simulink model "StateFlow_varB"  (R2022b)
settings: Solver=VariableStepAuto  StartTime=0.0  StopTime=500  FixedStep=0.001  RelTol=1e-3
InitFcn:
  | State_Flow_varB_setting
values from neighbouring files (symbols this model uses):
  Acceptable_press_offset = 5    [State_Flow_varB_setting.m]
  Desired_pressure_in_oxidiser_tank = 40    [State_Flow_varB_setting.m]
  Desired_pressure_in_pressure_section1 = 150    [State_Flow_varB_setting.m]
  Desired_pressure_in_pressure_section2 = 180    [State_Flow_varB_setting.m]
  s = struct    [State_Flow_varB_setting.m]
  Servo_open_limit = 20    [State_Flow_varB_setting.m]
  UDP_FC_send_packet_length = 68    [State_Flow_varB_setting.m]
  UDP_FC_send_sample_time = 0.05    [State_Flow_varB_setting.m]
  UDP_GSE_Curr_loop_receive_sample_time = 0.01    [State_Flow_varB_setting.m]
  UDP_GSE_IO_send_sample_time = 0.05    [State_Flow_varB_setting.m]
  UDP_GSE_send_packet_length = 68    [State_Flow_varB_setting.m]
libraries: simulink x36, slrealtimeiplib x16, slpidlib x6
(part 1 of 3)
settings Model: Creator=START  LastModifiedBy=START
settings DataIOCC: FinalStateName=xInitial  InitialState=SAVE  SaveOperatingPoint=on

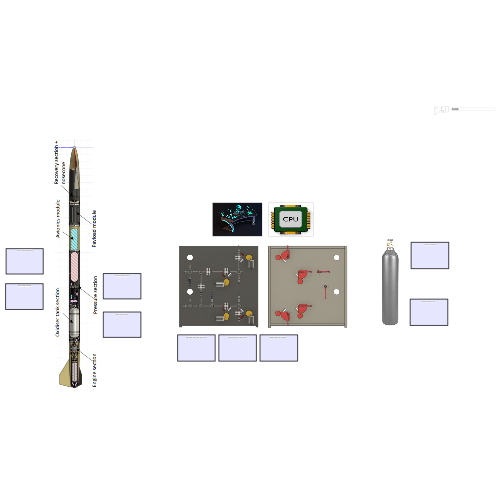
[thumbnail: Simulink's stored preview of the top-level diagram]
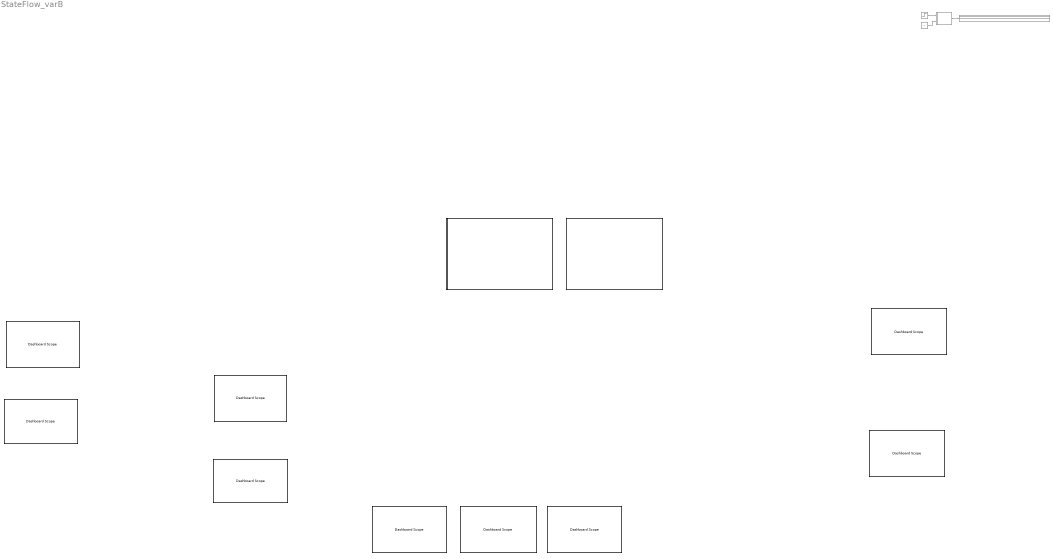
== system StateFlow_varB ==
  note: N2 bomb pressure level
  note: Rocket releasing valve state
  note: Rocket venting valve state
  note: Main tank pressure level
  note: Pressure section pressure level
  note: GSE N2 Releasing valve reported
  note: GSE N2 fueling valve state reported
  note: GSE Oxidiser fueling valve state reported
  note: N2O bomb pressure level
  Constant : Constant  Commented=on  Value=s  OutDataTypeStr=Bus: s_bus
  Dashboard Scope{,1,8,14} (4 alike) : DashboardScope  Ymin=0  Ymax=330
  Dashboard Scope11 : DashboardScope  Ymin=0  Ymax=260
  Dashboard Scope12 : DashboardScope  Ymin=0  Ymax=260
  Dashboard Scope13 : DashboardScope  Ymin=0  Ymax=260
  Dashboard Scope4 : DashboardScope  Ymin=0  Ymax=100
  Dashboard Scope6 : DashboardScope  Ymin=0  Ymax=90
  Display : Display  Commented=on
  MATLAB Function : MATLAB Function  Commented=on  TreatAsAtomicUnit=on
  Step : Step  Commented=on  SampleTime=0
  Subsystem4 : Subsystem
      mask Display: image('console4_1.jpg');
  Subsystem6 : Subsystem
      mask Display: image('CPU.png');
  wires:
  MATLAB Function/1(y) -> Display/1
  Step/1 -> MATLAB Function/1(u)
  Constant/1 -> MATLAB Function/2(inside)

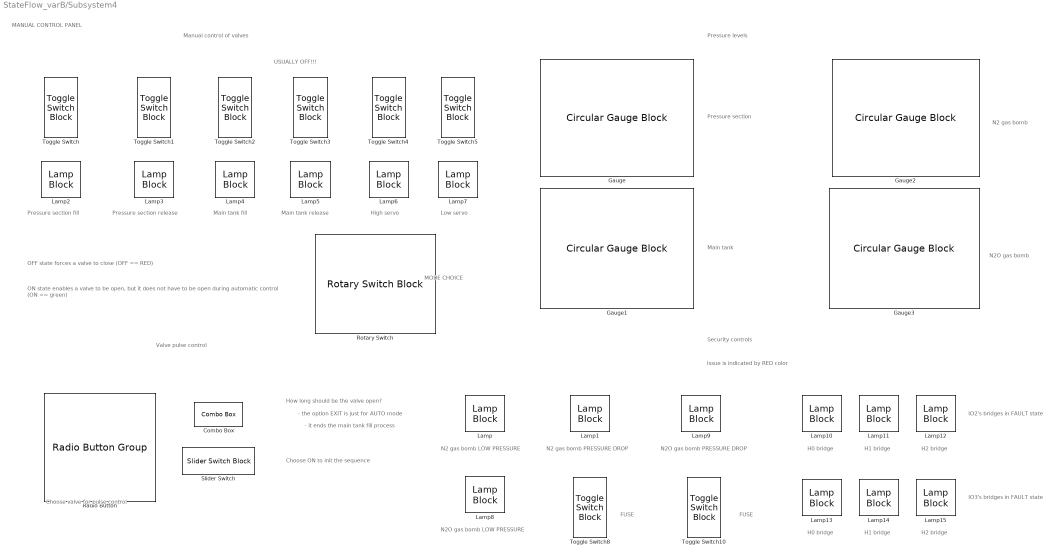
== system StateFlow_varB/Subsystem4 ==
  note: USUALLY OFF!!!
  note: N2 gas bomb LOW PRESSURE
  note: MANUAL CONTROL PANEL
  note: How long should be the valve open?
  note: Pressure levels
  note: Pressure section
  note: Main tank
  note: N2O gas bomb
  note: N2 gas bomb
  note: Manual control of valves
  note: Pressure section fill
  note: Pressure section release
  note: Main tank fill
  note: Main tank release
  note: High servo
  note: Low servo
  note: MODE CHOICE
  note: Security controls
  note: N2 gas bomb PRESSURE DROP
  note: OFF state forces a valve to close (OFF == RED)
  note: ON state enables a valve to be open, but it does not have to be open during automatic control (ON == green)
  note: N2O gas bomb LOW PRESSURE
  note: N2O gas bomb PRESSURE DROP
  note: Issue is indicated by RED color
  note: H0 bridge
  note: Valve pulse control
  note: - the option EXIT is just for AUTO mode
  note: - it ends the main tank fill process
  note: Choose ON to init the sequence
  note: Choose valve for pulse control
  note: FUSE
  note: FUSE
  note: IO2's bridges in FAULT state
  note: H1 bridge
  note: H2 bridge
  note: H1 bridge
  note: H2 bridge
  note: H0 bridge
  note: IO3's bridges in FAULT state
  Combo Box : ComboBox  LabelPosition=Hide  SelectedLabel=Exit
      settings: Values={{'0.5 s', '1 s', '2 s', '5 s', '10 s', 'Exit'}, [0 1 2 5 10 1000]}
  Gauge : CircularGaugeBlock  ScaleMax=300
  Gauge1 : CircularGaugeBlock
  Gauge2 : CircularGaugeBlock  ScaleMax=300
  Gauge3 : CircularGaugeBlock  ScaleMax=300
  Lamp{,1..15} (16 alike) : LampBlock  LabelPosition=Hide
  Radio Button : RadioButtonGroup  SelectedLabel=Main tank fill  ButtonGroupName=Valves
      settings: Values={{'Pressure section fill', 'Pressure section release', 'Main tank fill', 'Main tank release', 'High servo', 'Low servo'}, [0 1 2 3 4 5]}
  Rotary Switch : RotarySwitchBlock
      settings: Values={{'OFF', 'MAN', 'AUTO'}, [0 1 2]}
  Slider Switch : SliderSwitchBlock
      settings: Values={{'OFF', 'ON'}, [0 1]}
  Toggle Switch{,1..5,8,10} (8 alike) : ToggleSwitchBlock
      settings: Values={{'Off', 'On'}, [0 1]}

== system StateFlow_varB/Subsystem6 ==
  AND : Logic  IconShape=distinctive  AllPortsSameDT=off  OutDataTypeStr=boolean
  Chart : Stateflow chart  TreatAsAtomicUnit=on
  Compare To Constant : simulink/Logic and Bit Operations/Compare To Constant  relop===  const=1  OutDataTypeStr=boolean
  Compare To Constant1 : simulink/Logic and Bit Operations/Compare To Constant  relop===  const=2  OutDataTypeStr=boolean
  Constant : Constant  Value=2
  Constant1 : Constant
  Constant2 : Constant  Value=2
  Constant3 : Constant  Value=1000
  OR : Logic  Operator=OR  IconShape=distinctive  AllPortsSameDT=off  OutDataTypeStr=boolean
  Subsystem : Subsystem
  Subsystem1 : Subsystem
  Subsystem10 : Subsystem
  Subsystem2 : Subsystem
  Subsystem3 : Subsystem
  wires:
  Chart/1(AUTO_STATE) -> Subsystem/Enable
  Chart/2(MAN_STATE) -> Subsystem10/Enable
  Chart/3(OFF_STATE) -> Subsystem1/Enable
  Constant/1 -> Compare To Constant/1, Chart/1(CNTRL)
  Subsystem3/1(Output1) -> Subsystem/1(Input)
  Subsystem3/2(Input1) -> Subsystem/2(Input1)
  Subsystem3/3(Input2) -> Subsystem/3(Input2)
  Subsystem3/4(Input3) -> Subsystem/4(Input3)
  Subsystem3/5(Output) -> Subsystem/5(Input4)
  AND/1 -> Subsystem2/Enable
  OR/1 -> AND/1
  Constant1/1 -> Subsystem/7(Input6), AND/2
  Compare To Constant/1 -> OR/1
  Constant2/1 -> Subsystem2/1(Input), Compare To Constant1/1
  Compare To Constant1/1 -> OR/2
  Constant3/1 -> Subsystem/6(Input5), Subsystem2/2(Input1)

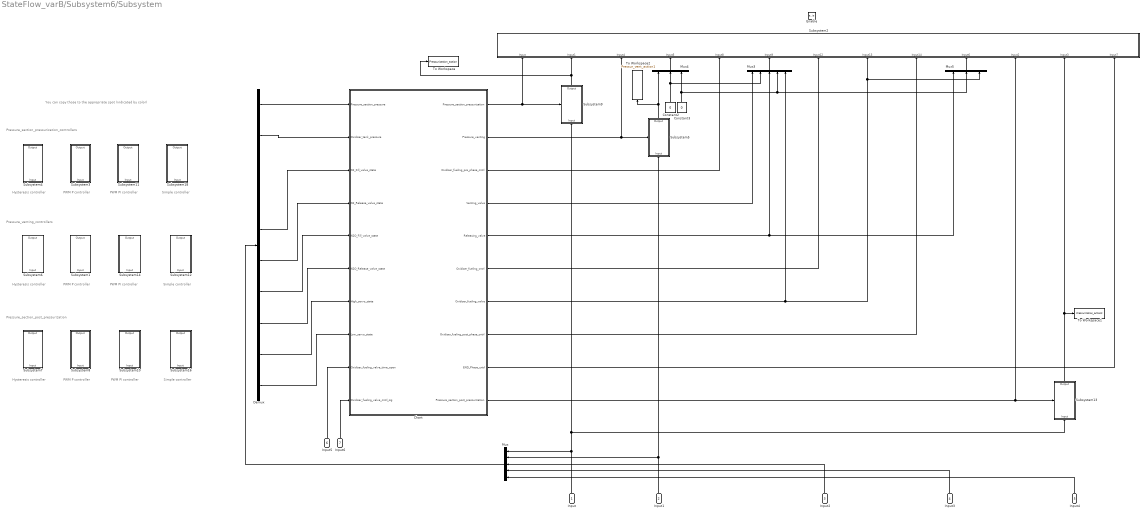
== system StateFlow_varB/Subsystem6/Subsystem ==
  note: You can copy those to the appropriate spot (indicated by color)
  note: Hysteresis controller
  note: Pressure_section_pressurization_controllers
  note: Hysteresis controller
  note: Pressure_venting_controllers
  note: Pressure_section_post_pressurization
  note: Hysteresis controller
  note: PWM P controller
  note: PWM P controller
  note: PWM PI controller
  note: PWM PI controller
  note: PWM P controller
  note: PWM PI controller
  note: Simple controller
  note: Simple controller
  note: Simple controller
  Input : Inport
  Input1 : Inport  Port=2
  Input2 : Inport  Port=3
  Input3 : Inport  Port=4
  Input4 : Inport  Port=5
  Input5 : Inport  Port=6
  Input6 : Inport  Port=7
  Enable : EnablePort  StatesWhenEnabling=reset
  Chart : Stateflow chart  TreatAsAtomicUnit=on
  Constant2 : Constant  Value=0
  Constant3 : Constant  Value=0
  Demux : Demux  Outputs=10
  Mux : Mux  Inputs=5
  Mux3 : Mux  Inputs=5
  Mux4 : Mux  Inputs=3
  Mux5 : Mux  Inputs=3
  Subsystem1 : Subsystem
  Subsystem10 : Subsystem
  Subsystem11 : Subsystem
  Subsystem12 : Subsystem
  Subsystem13 : Subsystem
  Subsystem14 : Subsystem
  Subsystem16 : Subsystem
  Subsystem18 : Subsystem
  Subsystem2 : Subsystem
  Subsystem3 : Subsystem
  Subsystem4 : Subsystem
  Subsystem5 : Subsystem
  Subsystem6 : Subsystem
  Subsystem7 : Subsystem
  Subsystem8 : Subsystem
  Subsystem9 : Subsystem
  To Workspace : ToWorkspace  VariableName=Pressurization_action  SaveFormat=Timeseries  SampleTime=-1
  To Workspace1 : ToWorkspace  VariableName=Pressurization_action2  SaveFormat=Timeseries  SampleTime=-1
  To Workspace2 : ToWorkspace  VariableName=Pressur_vent_action1  SaveFormat=Structure With Time  SampleTime=-1
  wires:
  Mux3/1 -> Subsystem2/6(Input9)
  Demux/10 -> Chart/8(Low_servo_state)
  Chart/7(Oxidiser_fueling_valve) -> Mux5/3, Subsystem2/8(Input13), Mux3/5
  Constant3/1 -> Mux5/2, Mux3/4, Mux4/3
  Chart/6(Oxidiser_fueling_cntrl) -> Subsystem2/7(Input12)
  Chart/3(Oxidiser_fueling_pre_phase_cntrl) -> Subsystem2/5(Input8)
  Input5/1 -> Chart/9(Oxidiser_fueling_valve_time_open)
  Demux/5 -> Chart/3(N2_Fill_valve_state)
  Chart/4(Venting_valve) -> Mux3/1
  Mux4/1 -> Subsystem2/4(Input5)
  Input/1 -> Mux/1, Subsystem13/1(Input), Subsystem9/1(Input)
  Constant2/1 -> Mux3/2, Mux4/2
  Input1/1 -> Subsystem5/1(Input), Mux/2
  Chart/2(Pressure_venting) -> Subsystem5/Enable, Subsystem2/3(Input4)
  Chart/5(Releasing_valve) -> Mux5/1, Mux3/3
  Subsystem9/1(Output) -> To Workspace/1, Subsystem2/2(Input1)
  Demux/1 -> Chart/1(Pressure_section_pressure)
  Input6/1 -> Chart/10(Oxidiser_fueling_valve_cntrl_sig)
  Mux/1 -> Demux/1
  Demux/2 -> Chart/2(Oxidiser_tank_pressure)
  Mux5/1 -> Subsystem2/10(Input6)
  Demux/7 -> Chart/5(N2O_Fill_valve_state)
  Demux/6 -> Chart/4(N2_Release_valve_state)
  Demux/9 -> Chart/7(High_servo_state)
  Demux/8 -> Chart/6(N2O_Release_valve_state)
  Subsystem5/1(Output) -> To Workspace2/1, Mux4/1
  Chart/8(Oxidiser_fueling_post_phase_cntrl) -> Subsystem2/9(Input14)
  Chart/9(END_Phase_cntrl) -> Subsystem2/13(Input7)
  Subsystem13/1(Output) -> To Workspace1/1, Subsystem2/12(Input3)
  Input2/1 -> Mux/3
  Input3/1 -> Mux/4
  Input4/1 -> Mux/5
  Chart/1(Pressure_section_pressurization) -> Subsystem9/Enable, Subsystem2/1(Input)
  Chart/10(Pressure_section_post_pressurization) -> Subsystem13/Enable, Subsystem2/11(Input2)

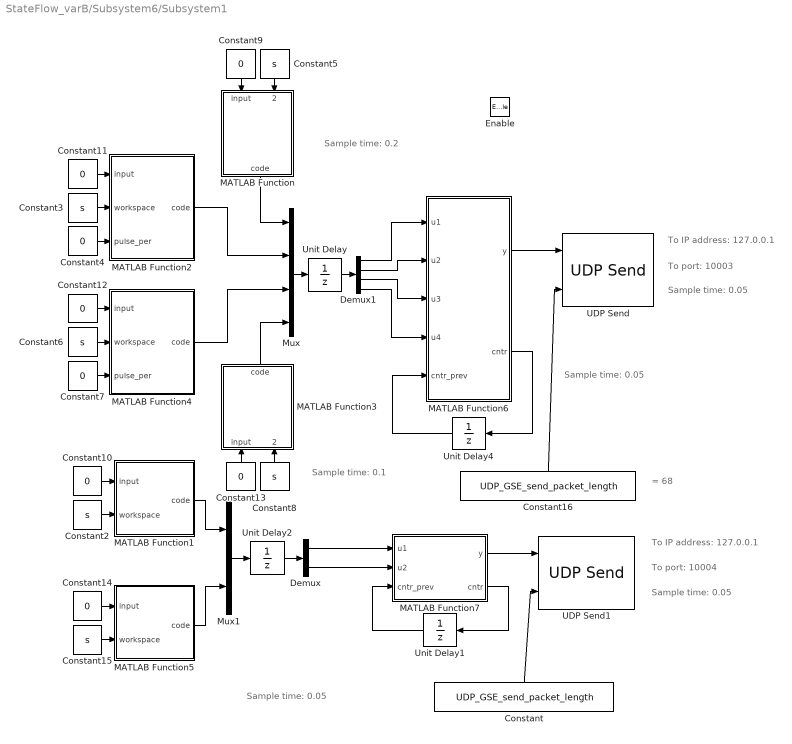
== system StateFlow_varB/Subsystem6/Subsystem1 ==
  note: To IP address: 127.0.0.1
  note: To port: 10003
  note: Sample time: 0.05
  note: To port: 10004
  note: To IP address: 127.0.0.1
  note: Sample time: 0.05
  note: = 68
  note: Sample time: 0.2
  note: Sample time: 0.05
  note: Sample time: 0.1
  note: Sample time: 0.05
  Enable : EnablePort  StatesWhenEnabling=reset
  Constant : Constant  Value=UDP_GSE_send_packet_length
  Constant{4,7,9..14} (8 alike) : Constant  Value=0
  Constant{2..3,5..6,8,15} (6 alike) : Constant  Value=s  OutDataTypeStr=Bus: s_bus
  Constant16 : Constant  Value=UDP_GSE_send_packet_length
  Demux : Demux  Outputs=2
  Demux1 : Demux
  MATLAB Function : MATLAB Function  TreatAsAtomicUnit=on
  MATLAB Function1 : MATLAB Function  TreatAsAtomicUnit=on
  MATLAB Function2 : MATLAB Function  TreatAsAtomicUnit=on
  MATLAB Function3 : MATLAB Function  TreatAsAtomicUnit=on
  MATLAB Function4 : MATLAB Function  TreatAsAtomicUnit=on
  MATLAB Function5 : MATLAB Function  TreatAsAtomicUnit=on
  MATLAB Function6 : MATLAB Function  TreatAsAtomicUnit=on
  MATLAB Function7 : MATLAB Function  TreatAsAtomicUnit=on
  Mux : Mux
  Mux1 : Mux  Inputs=2
  UDP Send : slrealtimeiplib/UDP Send  useHostTargetConn=off  toAddress=UDP_GSE_send_to_IP  toPort=IO_card_2_port  sampleTime=UDP_GSE_IO_send_sample_time  enableMessage=off
  UDP Send1 : slrealtimeiplib/UDP Send  useHostTargetConn=off  toAddress=UDP_GSE_send_to_IP  toPort=IO_card_3_port  sampleTime=UDP_GSE_IO_send_sample_time  enableMessage=off
  Unit Delay : UnitDelay  SampleTime=UDP_GSE_IO_send_sample_time*4  HasFrameUpgradeWarning=on
  Unit Delay1 : UnitDelay  InitialCondition=1  SampleTime=UDP_GSE_IO_send_sample_time  HasFrameUpgradeWarning=on
  Unit Delay2 : UnitDelay  SampleTime=UDP_GSE_IO_send_sample_time*2  HasFrameUpgradeWarning=on
  Unit Delay4 : UnitDelay  InitialCondition=1  SampleTime=UDP_GSE_IO_send_sample_time  HasFrameUpgradeWarning=on
  wires:
  Constant2/1 -> MATLAB Function1/2(workspace)
  Constant6/1 -> MATLAB Function4/2(workspace)
  Constant3/1 -> MATLAB Function2/2(workspace)
  Constant8/1 -> MATLAB Function3/2(workspace)
  Constant4/1 -> MATLAB Function2/3(pulse_per)
  Constant7/1 -> MATLAB Function4/3(pulse_per)
  Constant10/1 -> MATLAB Function1/1(input)
  Constant11/1 -> MATLAB Function2/1(input)
  Constant12/1 -> MATLAB Function4/1(input)
  Constant13/1 -> MATLAB Function3/1(input)
  Constant14/1 -> MATLAB Function5/1(input)
  Constant15/1 -> MATLAB Function5/2(workspace)
  Constant16/1 -> UDP Send/2
  MATLAB Function1/1(code) -> Mux1/1
  MATLAB Function5/1(code) -> Mux1/2
  Constant/1 -> UDP Send1/2
  Mux/1 -> Unit Delay/1
  MATLAB Function/1(code) -> Mux/1
  MATLAB Function2/1(code) -> Mux/2
  MATLAB Function4/1(code) -> Mux/3
  MATLAB Function3/1(code) -> Mux/4
  Mux1/1 -> Unit Delay2/1
  MATLAB Function7/2(cntr) -> Unit Delay1/1
  Unit Delay1/1 -> MATLAB Function7/3(cntr_prev)
  MATLAB Function7/1(y) -> UDP Send1/1
  Unit Delay2/1 -> Demux/1
  Demux/1 -> MATLAB Function7/1(u1)
  Demux/2 -> MATLAB Function7/2(u2)
  Unit Delay/1 -> Demux1/1
  Demux1/4 -> MATLAB Function6/4(u4)
  Demux1/3 -> MATLAB Function6/3(u3)
  MATLAB Function6/2(cntr) -> Unit Delay4/1
  Demux1/1 -> MATLAB Function6/1(u1)
  Unit Delay4/1 -> MATLAB Function6/5(cntr_prev)
  Demux1/2 -> MATLAB Function6/2(u2)
  MATLAB Function6/1(y) -> UDP Send/1
  Constant5/1 -> MATLAB Function/2(workspace)
  Constant9/1 -> MATLAB Function/1(input)

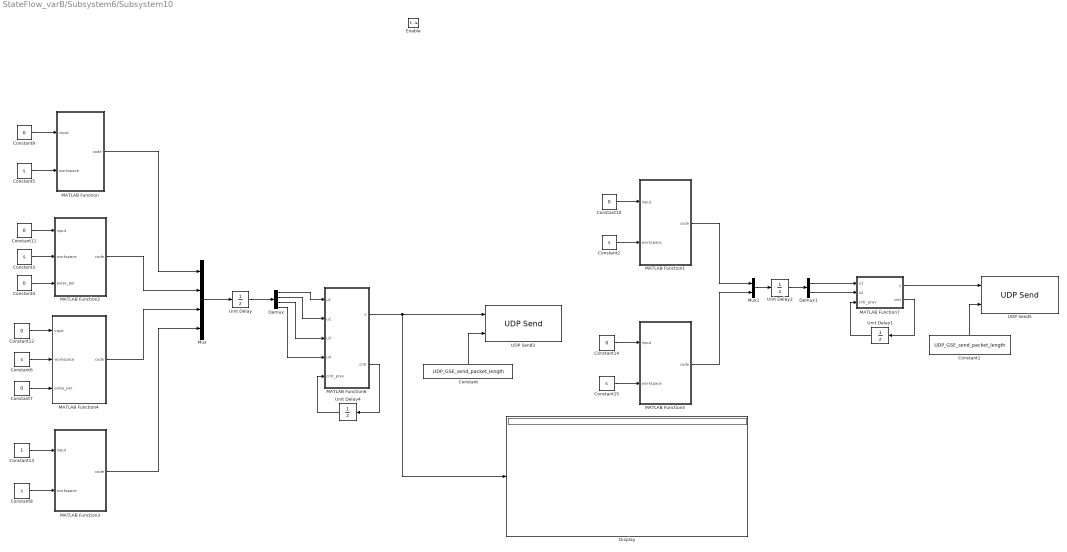
== system StateFlow_varB/Subsystem6/Subsystem10 ==
  Enable : EnablePort  StatesWhenEnabling=reset
  Constant : Constant  Value=UDP_GSE_send_packet_length
  Constant1 : Constant  Value=UDP_GSE_send_packet_length
  Constant{4,7,9..12,14} (7 alike) : Constant  Value=0
  Constant13 : Constant
  Constant{2..3,5..6,8,15} (6 alike) : Constant  Value=s  OutDataTypeStr=Bus: s_bus
  Demux : Demux
  Demux1 : Demux  Outputs=2
  Display : Display
  MATLAB Function : MATLAB Function  TreatAsAtomicUnit=on
  MATLAB Function1 : MATLAB Function  TreatAsAtomicUnit=on
  MATLAB Function2 : MATLAB Function  TreatAsAtomicUnit=on
  MATLAB Function3 : MATLAB Function  TreatAsAtomicUnit=on
  MATLAB Function4 : MATLAB Function  TreatAsAtomicUnit=on
  MATLAB Function5 : MATLAB Function  TreatAsAtomicUnit=on
  MATLAB Function6 : MATLAB Function  TreatAsAtomicUnit=on
  MATLAB Function7 : MATLAB Function  TreatAsAtomicUnit=on
  Mux : Mux
  Mux1 : Mux  Inputs=2
  UDP Send3 : slrealtimeiplib/UDP Send  useHostTargetConn=off  toAddress=UDP_GSE_send_to_IP  toPort=IO_card_2_port  sampleTime=UDP_GSE_IO_send_sample_time  enableMessage=off
  UDP Send5 : slrealtimeiplib/UDP Send  useHostTargetConn=off  toAddress=UDP_GSE_send_to_IP  toPort=IO_card_3_port  sampleTime=UDP_GSE_IO_send_sample_time  enableMessage=off
  Unit Delay : UnitDelay  SampleTime=UDP_GSE_IO_send_sample_time*4  HasFrameUpgradeWarning=on
  Unit Delay1 : UnitDelay  InitialCondition=1  SampleTime=UDP_GSE_IO_send_sample_time  HasFrameUpgradeWarning=on
  Unit Delay2 : UnitDelay  SampleTime=UDP_GSE_IO_send_sample_time*2  HasFrameUpgradeWarning=on
  Unit Delay4 : UnitDelay  InitialCondition=1  SampleTime=UDP_GSE_IO_send_sample_time  HasFrameUpgradeWarning=on
  wires:
  Constant2/1 -> MATLAB Function1/2(workspace)
  Constant6/1 -> MATLAB Function4/2(workspace)
  Constant3/1 -> MATLAB Function2/2(workspace)
  Constant8/1 -> MATLAB Function3/2(workspace)
  Constant4/1 -> MATLAB Function2/3(pulse_per)
  Constant7/1 -> MATLAB Function4/3(pulse_per)
  Constant10/1 -> MATLAB Function1/1(input)
  Constant11/1 -> MATLAB Function2/1(input)
  Constant12/1 -> MATLAB Function4/1(input)
  Constant13/1 -> MATLAB Function3/1(input)
  Constant14/1 -> MATLAB Function5/1(input)
  Constant15/1 -> MATLAB Function5/2(workspace)
  MATLAB Function/1(code) -> Mux/1
  Constant5/1 -> MATLAB Function/2(workspace)
  Constant9/1 -> MATLAB Function/1(input)
  MATLAB Function2/1(code) -> Mux/2
  MATLAB Function4/1(code) -> Mux/3
  MATLAB Function3/1(code) -> Mux/4
  Mux/1 -> Unit Delay/1
  MATLAB Function1/1(code) -> Mux1/1
  MATLAB Function5/1(code) -> Mux1/2
  Mux1/1 -> Unit Delay2/1
  Unit Delay/1 -> Demux/1
  Demux/4 -> MATLAB Function6/4(u4)
  Demux/3 -> MATLAB Function6/3(u3)
  MATLAB Function6/2(cntr) -> Unit Delay4/1
  Demux/1 -> MATLAB Function6/1(u1)
  Unit Delay4/1 -> MATLAB Function6/5(cntr_prev)
  Demux/2 -> MATLAB Function6/2(u2)
  Unit Delay2/1 -> Demux1/1
  MATLAB Function7/2(cntr) -> Unit Delay1/1
  Demux1/1 -> MATLAB Function7/1(u1)
  Unit Delay1/1 -> MATLAB Function7/3(cntr_prev)
  Demux1/2 -> MATLAB Function7/2(u2)
  MATLAB Function6/1(y) -> Display/1, UDP Send3/1
  Constant/1 -> UDP Send3/2
  MATLAB Function7/1(y) -> UDP Send5/1
  Constant1/1 -> UDP Send5/2

== system StateFlow_varB/Subsystem6/Subsystem2 ==
  Input : Inport
  Input1 : Inport  Port=2
  Enable : EnablePort  StatesWhenEnabling=reset
  MATLAB Function : MATLAB Function  TreatAsAtomicUnit=on
  Unit Delay : UnitDelay  SampleTime=0.05  HasFrameUpgradeWarning=on
  wires:
  Input/1 -> MATLAB Function/1(valve)
  Input1/1 -> MATLAB Function/2(time_des)
  MATLAB Function/1(time_curr) -> Unit Delay/1
  Unit Delay/1 -> MATLAB Function/3(time_curr1)

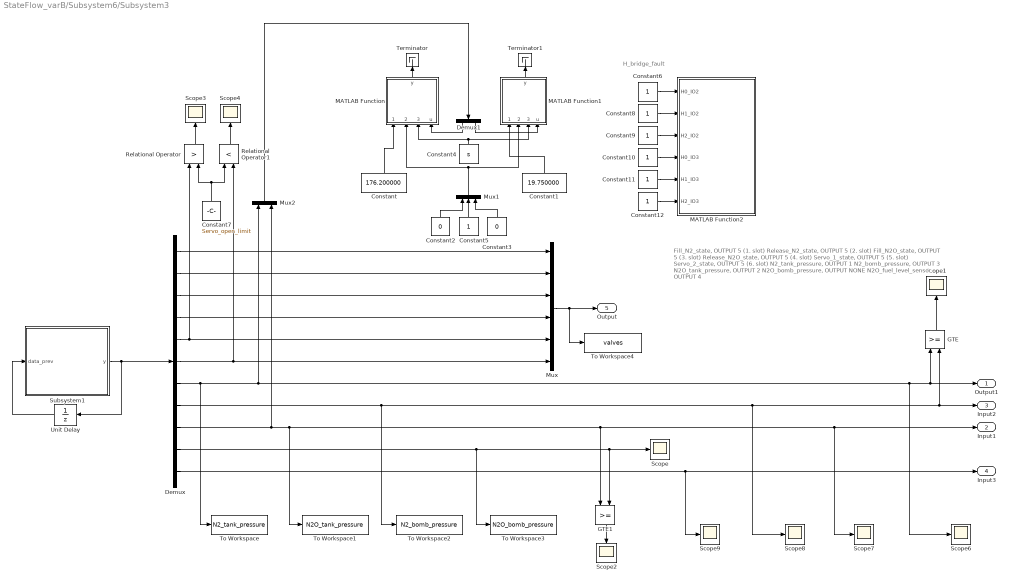
== system StateFlow_varB/Subsystem6/Subsystem3 ==
  note: H_bridge_fault
  note: Fill_N2_state, OUTPUT 5 (1. slot)
      | Release_N2_state, OUTPUT 5 (2. slot)
      | Fill_N2O_state, OUTPUT 5 (3. slot)
      | Release_N2O_state, OUTPUT 5 (4. slot)
      | Servo_1_state, OUTPUT 5 (5. slot)
      | Servo_2_state, OUTPUT 5 (6. slot)
      | N2_tank_pressure, OUTPUT 1
      | N2_bomb_pressure, OUTPUT 3
      | N2O_tank_pressure, OUTPUT 2
      | N2O_bomb_pressure, OUTPUT NONE
      | N2O_fuel_level_sensor OUTPUT 4
  Constant : Constant  Value=176.200000
  Constant1 : Constant  Value=19.750000
  Constant{5..6,8..12} (7 alike) : Constant
  Constant2 : Constant  Value=0
  Constant3 : Constant  Value=0
  Constant4 : Constant  Value=s  OutDataTypeStr=Bus: s_bus
  Constant7 : Constant  Value=Servo_open_limit
  Demux : Demux  Outputs=11
  Demux1 : Demux  Outputs=2
  GTE : RelationalOperator  OutDataTypeStr=boolean  RndMeth=Simplest  InputSameDT=off
  GTE1 : RelationalOperator  OutDataTypeStr=boolean  RndMeth=Simplest  InputSameDT=off
  MATLAB Function : MATLAB Function  TreatAsAtomicUnit=on
  MATLAB Function1 : MATLAB Function  TreatAsAtomicUnit=on
  MATLAB Function2 : MATLAB Function  TreatAsAtomicUnit=on
  Mux : Mux  Inputs=6
  Mux1 : Mux  Inputs=3
  Mux2 : Mux  Inputs=2
  Relational Operator : RelationalOperator  Operator=>  OutDataTypeStr=boolean  RndMeth=Simplest  InputSameDT=off
  Relational Operator1 : RelationalOperator  Operator=<  OutDataTypeStr=boolean  RndMeth=Simplest  InputSameDT=off
  Scope{,1..4,6..9} (9 alike) : Scope
  Subsystem1 : Subsystem
  Terminator : Terminator
  Terminator1 : Terminator
  To Workspace : ToWorkspace  VariableName=N2_tank_pressure  SaveFormat=Structure With Time  SampleTime=-1
  To Workspace1 : ToWorkspace  VariableName=N2O_tank_pressure  SaveFormat=Structure With Time  SampleTime=-1
  To Workspace2 : ToWorkspace  VariableName=N2_bomb_pressure  SaveFormat=Structure With Time  SampleTime=-1
  To Workspace3 : ToWorkspace  VariableName=N2O_bomb_pressure  SaveFormat=Structure With Time  SampleTime=-1
  To Workspace4 : ToWorkspace  VariableName=valves  SaveFormat=Structure With Time  SampleTime=-1
  Unit Delay : UnitDelay  SampleTime=-1  HasFrameUpgradeWarning=on
  Output1 : Outport
  Input1 : Outport  Port=2
  Input2 : Outport  Port=3
  Input3 : Outport  Port=4
  Output : Outport  Port=5
  wires:
  Subsystem1/1(y) -> Unit Delay/1, Demux/1
  Demux/7 -> To Workspace/1, Mux2/1, GTE/1, Output1/1, Scope6/1
  Demux/11 -> Scope9/1, Input3/1
  Demux/9 -> Mux2/2, To Workspace1/1, GTE1/1, Scope7/1, Input1/1
  Demux/8 -> To Workspace2/1, Scope8/1, GTE/2, Input2/1
  Demux/6 -> Relational Operator1/2, Mux/6
  Demux/5 -> Relational Operator/1, Mux/5
  Demux/4 -> Mux/4
  Demux/3 -> Mux/3
  Demux/2 -> Mux/2
  Demux/1 -> Mux/1
  Mux/1 -> To Workspace4/1, Output/1
  Unit Delay/1 -> Subsystem1/1(data_prev)
  Demux/10 -> To Workspace3/1, GTE1/2, Scope/1
  GTE/1 -> Scope1/1
  GTE1/1 -> Scope2/1
  Constant4/1 -> MATLAB Function/3(workspace), MATLAB Function1/3(workspace)
  MATLAB Function/1(y) -> Terminator/1
  Demux1/1 -> MATLAB Function/4(u)
  Constant/1 -> MATLAB Function/1(val_const)
  MATLAB Function1/1(y) -> Terminator1/1
  Mux1/1 -> MATLAB Function1/2(valves_state), MATLAB Function/2(valves_state)
  Demux1/2 -> MATLAB Function1/4(u)
  Constant1/1 -> MATLAB Function1/1(val_const)
  Constant2/1 -> Mux1/1
  Mux2/1 -> Demux1/1
  Constant5/1 -> Mux1/2
  Constant3/1 -> Mux1/3
  Constant6/1 -> MATLAB Function2/1(H0_IO2)
  Constant7/1 -> Relational Operator/2, Relational Operator1/1
  Relational Operator/1 -> Scope3/1
  Relational Operator1/1 -> Scope4/1
  Constant8/1 -> MATLAB Function2/2(H1_IO2)
  Constant9/1 -> MATLAB Function2/3(H2_IO2)
  Constant10/1 -> MATLAB Function2/4(H0_IO3)
  Constant11/1 -> MATLAB Function2/5(H1_IO3)
  Constant12/1 -> MATLAB Function2/6(H2_IO3)

== system StateFlow_varB/Subsystem6/Subsystem/Subsystem1 ==
  Input : Inport
  Enable : EnablePort
  Constant : Constant  Value=Desired_pressure_in_oxidiser_tank
  Constant1 : Constant  Commented=on  Value=s  OutDataTypeStr=Bus: s_bus
  Gain7 : Gain  Gain=-1
  MATLAB Function : MATLAB Function  Commented=on  TreatAsAtomicUnit=on
  Mux : Mux  Inputs=2
  PID Controller6 : slpidlib/PID Controller  Controller=PID  Form=Parallel  TimeDomain=Discrete-time  UseExternalTs=off  SampleTime=-1  IntegratorMethod=Forward Euler  FilterMethod=Forward Euler  ControllerParametersSource=internal  P=0.0077  I=0  UseKiTs=off  D=0  N=0  UseFilter=on  TunerSelectOption=Transfer Function Based (PID Tuner App)  InitialConditionSource=internal  InitialConditionForIntegrator=0  InitialConditionForFilter=0  DifferentiatorICPrevScaledInput=0  ExternalReset=none  TrackingMode=off  Kt=1  LimitOutput=on  SatLimitsSource=internal  UpperSaturationLimit=1  LowerSaturationLimit=-1  LinearizeAsGain=on  AntiWindupMode=clamping  Kb=1  LimitIntegrator=off  UpperIntegratorSaturationLimit=0.05  LowerIntegratorSaturationLimit=-inf  POutMin=[]  POutMax=[]  IOutMin=[]  IOutMax=[]  DOutMin=[]  DOutMax=[]  NOutMin=[]  NOutMax=[]  SumOutMin=[]  SumOutMax=[]  SaturationOutMin=[]  SaturationOutMax=[]  PParamMin=[]  PParamMax=[]  IParamMin=[]  IParamMax=[]  DParamMin=[]  DParamMax=[]  NParamMin=[]  NParamMax=[]  KbParamMin=[]  KbParamMax=[]  KtParamMin=[]  KtParamMax=[]  KbOutMin=[]  KbOutMax=[]  KtOutMin=[]  KtOutMax=[]  IntegratorOutMin=[]  IntegratorOutMax=[]  FilterOutMin=[]  FilterOutMax=[]  SumI1OutMin=[]  SumI1OutMax=[]  SumI2OutMin=[]  SumI2OutMax=[]  SumI3OutMin=[]  SumI3OutMax=[]  SumI4OutMin=[]  SumI4OutMax=[]  SumDOutMin=[]  SumDOutMax=[]  DifferentiatorOutMin=[]  DifferentiatorOutMax=[]  FilterDiffOutCoefMin=[]  FilterDiffOutCoefMax=[]  ReciprocalOutMin=[]  ReciprocalOutMax=[]  SumDenOutMin=[]  SumDenOutMax=[]  SumNumOutMin=[]  SumNumOutMax=[]  DivideOutMin=[]  DivideOutMax=[]  UdiffTsProdOutMin=[]  UdiffTsProdOutMax=[]  NTsProdOutMin=[]  NTsProdOutMax=[]  UintegralTsProdOutMin=[]  UintegralTsProdOutMax=[]  UngainTsProdOutMin=[]  UngainTsProdOutMax=[]  ClampingZeroOutDataTypeStr=Inherit: Inherit via back propagation  ClampingZeroOutMin=[]  ClampingZeroOutMax=[]  FilterDenConstantOutDataTypeStr=Inherit: Inherit via back propagation  FilterDenConstantOutMin=[]  FilterDenConstantOutMax=[]  PCopyOutDataTypeStr=Inherit: Inherit via back propagation  PCopyOutMin=[]  PCopyOutMax=[]  NCopyOutDataTypeStr=Inherit: Inherit via back propagation  NCopyOutMin=[]  NCopyOutMax=[]  IntegratorContinuousStateAttributes=''  IntegratorStateMustResolveToSignalObject=off  IntegratorRTWStateStorageClass=Auto  FilterContinuousStateAttributes=''  FilterStateMustResolveToSignalObject=off  FilterRTWStateStorageClass=Auto  ParallelPVariant=InternalParameters  IdealPVariant=Disabled  IVariant=InternalParameters  DVariant=InternalParameters  IntegratorVariant=Discrete  SatVariant=Enabled  AWVariant=DiscClampingParallel  PCopyVariant=Disabled  TRVariant=Disabled  FdbkBlocksVariant=Forward  IdealPFdbkVariant=Disabled  SatFdbkVariant=Disabled  DerivativeFilterVariant=ForwardEulerFilter  NVariant=InternalParameters  NCopyVariant=Disabled  FilterICVariant=InternalICsFilter  IntegratorICVariant=InternalICs  ExternalResetVariant=Disabled  TRSumVariant=Passthrough  SumFdbkVariant=Disabled  SumVariant=Sum_PID  TsampFilterVariant=InternalTs  TsampNgainVariant=Passthrough  TsampIntegralVariant=Passthrough  ExternalSaturationOutDataTypeStr=Inherit: Same as second input
  PWM : simulink/Discontinuities/PWM  DisableCoverage=on  Period=2  InitialDelay=0  DisallowZeroDutyCycle=off  RunAtFixedTimeIntervals=off  SampleTime=0.1
  PWM1 : simulink/Discontinuities/PWM  DisableCoverage=on  Period=2  InitialDelay=0  DisallowZeroDutyCycle=off  RunAtFixedTimeIntervals=off  SampleTime=0.1
  Sum8 : Sum  Inputs=|+-
  Terminator : Terminator  Commented=on
  Output : Outport
  wires:
  Constant/1 -> Sum8/1
  Sum8/1 -> PID Controller6/1
  PID Controller6/1 -> PWM/1, Gain7/1
  Gain7/1 -> PWM1/1
  Mux/1 -> Output/1
  Input/1 -> Sum8/2
  MATLAB Function/1(y) -> Terminator/1
  Constant1/1 -> MATLAB Function/3(workspace)
  PWM/1 -> Mux/1
  PWM1/1 -> Mux/2

== system StateFlow_varB/Subsystem6/Subsystem/Subsystem10 ==
  Input : Inport
  Enable : EnablePort
  Constant : Constant  Value=Desired_pressure_in_pressure_section1
  Gain4 : Gain  Gain=-1
  Mux : Mux  Inputs=2
  PID Controller5 : slpidlib/PID Controller  Controller=PID  Form=Parallel  TimeDomain=Discrete-time  UseExternalTs=off  SampleTime=-1  IntegratorMethod=Forward Euler  FilterMethod=Forward Euler  ControllerParametersSource=internal  P=0.0027  I=0.00002  UseKiTs=off  D=0  N=0  UseFilter=on  TunerSelectOption=Transfer Function Based (PID Tuner App)  InitialConditionSource=internal  InitialConditionForIntegrator=0  InitialConditionForFilter=0  DifferentiatorICPrevScaledInput=0  ExternalReset=none  TrackingMode=off  Kt=1  LimitOutput=on  SatLimitsSource=internal  UpperSaturationLimit=1  LowerSaturationLimit=-1  LinearizeAsGain=off  AntiWindupMode=clamping  Kb=1  LimitIntegrator=on  UpperIntegratorSaturationLimit=0.05  LowerIntegratorSaturationLimit=-0.05  POutMin=[]  POutMax=[]  IOutMin=[]  IOutMax=[]  DOutMin=[]  DOutMax=[]  NOutMin=[]  NOutMax=[]  SumOutMin=[]  SumOutMax=[]  SaturationOutMin=[]  SaturationOutMax=[]  PParamMin=[]  PParamMax=[]  IParamMin=[]  IParamMax=[]  DParamMin=[]  DParamMax=[]  NParamMin=[]  NParamMax=[]  KbParamMin=[]  KbParamMax=[]  KtParamMin=[]  KtParamMax=[]  KbOutMin=[]  KbOutMax=[]  KtOutMin=[]  KtOutMax=[]  IntegratorOutMin=[]  IntegratorOutMax=[]  FilterOutMin=[]  FilterOutMax=[]  SumI1OutMin=[]  SumI1OutMax=[]  SumI2OutMin=[]  SumI2OutMax=[]  SumI3OutMin=[]  SumI3OutMax=[]  SumI4OutMin=[]  SumI4OutMax=[]  SumDOutMin=[]  SumDOutMax=[]  DifferentiatorOutMin=[]  DifferentiatorOutMax=[]  FilterDiffOutCoefMin=[]  FilterDiffOutCoefMax=[]  ReciprocalOutMin=[]  ReciprocalOutMax=[]  SumDenOutMin=[]  SumDenOutMax=[]  SumNumOutMin=[]  SumNumOutMax=[]  DivideOutMin=[]  DivideOutMax=[]  UdiffTsProdOutMin=[]  UdiffTsProdOutMax=[]  NTsProdOutMin=[]  NTsProdOutMax=[]  UintegralTsProdOutMin=[]  UintegralTsProdOutMax=[]  UngainTsProdOutMin=[]  UngainTsProdOutMax=[]  ClampingZeroOutDataTypeStr=Inherit: Inherit via back propagation  ClampingZeroOutMin=[]  ClampingZeroOutMax=[]  FilterDenConstantOutDataTypeStr=Inherit: Inherit via back propagation  FilterDenConstantOutMin=[]  FilterDenConstantOutMax=[]  PCopyOutDataTypeStr=Inherit: Inherit via back propagation  PCopyOutMin=[]  PCopyOutMax=[]  NCopyOutDataTypeStr=Inherit: Inherit via back propagation  NCopyOutMin=[]  NCopyOutMax=[]  IntegratorContinuousStateAttributes=''  IntegratorStateMustResolveToSignalObject=off  IntegratorRTWStateStorageClass=Auto  FilterContinuousStateAttributes=''  FilterStateMustResolveToSignalObject=off  FilterRTWStateStorageClass=Auto  ParallelPVariant=InternalParameters  IdealPVariant=Disabled  IVariant=InternalParameters  DVariant=InternalParameters  IntegratorVariant=Discrete  SatVariant=Enabled  AWVariant=DiscClampingParallel  PCopyVariant=Disabled  TRVariant=Disabled  FdbkBlocksVariant=Forward  IdealPFdbkVariant=Disabled  SatFdbkVariant=Disabled  DerivativeFilterVariant=ForwardEulerFilter  NVariant=InternalParameters  NCopyVariant=Disabled  FilterICVariant=InternalICsFilter  IntegratorICVariant=InternalICs  ExternalResetVariant=Disabled  TRSumVariant=Passthrough  SumFdbkVariant=Disabled  SumVariant=Sum_PID  TsampFilterVariant=InternalTs  TsampNgainVariant=Passthrough  TsampIntegralVariant=Passthrough  ExternalSaturationOutDataTypeStr=Inherit: Same as second input
  PWM7 : simulink/Discontinuities/PWM  DisableCoverage=on  Period=2  InitialDelay=0  DisallowZeroDutyCycle=off  RunAtFixedTimeIntervals=off  SampleTime=0.1
  PWM8 : simulink/Discontinuities/PWM  DisableCoverage=on  Period=2  InitialDelay=0  DisallowZeroDutyCycle=off  RunAtFixedTimeIntervals=off  SampleTime=0.1
  Saturation13 : Saturate  UpperLimit=1  LowerLimit=0
  Saturation14 : Saturate  UpperLimit=1  LowerLimit=0
  Sum6 : Sum  Inputs=|+-
  Output : Outport
  wires:
  PID Controller5/1 -> Gain4/1, Saturation14/1
  Saturation13/1 -> PWM8/1
  Gain4/1 -> Saturation13/1
  Constant/1 -> Sum6/1
  Sum6/1 -> PID Controller5/1
  Saturation14/1 -> PWM7/1
  PWM8/1 -> Mux/2
  PWM7/1 -> Mux/1
  Mux/1 -> Output/1
  Input/1 -> Sum6/2

== system StateFlow_varB/Subsystem6/Subsystem/Subsystem11 ==
  Input : Inport
  Enable : EnablePort
  Constant : Constant  Value=Desired_pressure_in_pressure_section1
  Gain4 : Gain  Gain=-1
  Mux : Mux  Inputs=2
  PID Controller5 : slpidlib/PID Controller  Controller=PID  Form=Parallel  TimeDomain=Discrete-time  UseExternalTs=off  SampleTime=-1  IntegratorMethod=Forward Euler  FilterMethod=Forward Euler  ControllerParametersSource=internal  P=0.0027  I=0.00002  UseKiTs=off  D=0  N=0  UseFilter=on  TunerSelectOption=Transfer Function Based (PID Tuner App)  InitialConditionSource=internal  InitialConditionForIntegrator=0  InitialConditionForFilter=0  DifferentiatorICPrevScaledInput=0  ExternalReset=none  TrackingMode=off  Kt=1  LimitOutput=on  SatLimitsSource=internal  UpperSaturationLimit=1  LowerSaturationLimit=-1  LinearizeAsGain=off  AntiWindupMode=clamping  Kb=1  LimitIntegrator=on  UpperIntegratorSaturationLimit=0.05  LowerIntegratorSaturationLimit=-0.05  POutMin=[]  POutMax=[]  IOutMin=[]  IOutMax=[]  DOutMin=[]  DOutMax=[]  NOutMin=[]  NOutMax=[]  SumOutMin=[]  SumOutMax=[]  SaturationOutMin=[]  SaturationOutMax=[]  PParamMin=[]  PParamMax=[]  IParamMin=[]  IParamMax=[]  DParamMin=[]  DParamMax=[]  NParamMin=[]  NParamMax=[]  KbParamMin=[]  KbParamMax=[]  KtParamMin=[]  KtParamMax=[]  KbOutMin=[]  KbOutMax=[]  KtOutMin=[]  KtOutMax=[]  IntegratorOutMin=[]  IntegratorOutMax=[]  FilterOutMin=[]  FilterOutMax=[]  SumI1OutMin=[]  SumI1OutMax=[]  SumI2OutMin=[]  SumI2OutMax=[]  SumI3OutMin=[]  SumI3OutMax=[]  SumI4OutMin=[]  SumI4OutMax=[]  SumDOutMin=[]  SumDOutMax=[]  DifferentiatorOutMin=[]  DifferentiatorOutMax=[]  FilterDiffOutCoefMin=[]  FilterDiffOutCoefMax=[]  ReciprocalOutMin=[]  ReciprocalOutMax=[]  SumDenOutMin=[]  SumDenOutMax=[]  SumNumOutMin=[]  SumNumOutMax=[]  DivideOutMin=[]  DivideOutMax=[]  UdiffTsProdOutMin=[]  UdiffTsProdOutMax=[]  NTsProdOutMin=[]  NTsProdOutMax=[]  UintegralTsProdOutMin=[]  UintegralTsProdOutMax=[]  UngainTsProdOutMin=[]  UngainTsProdOutMax=[]  ClampingZeroOutDataTypeStr=Inherit: Inherit via back propagation  ClampingZeroOutMin=[]  ClampingZeroOutMax=[]  FilterDenConstantOutDataTypeStr=Inherit: Inherit via back propagation  FilterDenConstantOutMin=[]  FilterDenConstantOutMax=[]  PCopyOutDataTypeStr=Inherit: Inherit via back propagation  PCopyOutMin=[]  PCopyOutMax=[]  NCopyOutDataTypeStr=Inherit: Inherit via back propagation  NCopyOutMin=[]  NCopyOutMax=[]  IntegratorContinuousStateAttributes=''  IntegratorStateMustResolveToSignalObject=off  IntegratorRTWStateStorageClass=Auto  FilterContinuousStateAttributes=''  FilterStateMustResolveToSignalObject=off  FilterRTWStateStorageClass=Auto  ParallelPVariant=InternalParameters  IdealPVariant=Disabled  IVariant=InternalParameters  DVariant=InternalParameters  IntegratorVariant=Discrete  SatVariant=Enabled  AWVariant=DiscClampingParallel  PCopyVariant=Disabled  TRVariant=Disabled  FdbkBlocksVariant=Forward  IdealPFdbkVariant=Disabled  SatFdbkVariant=Disabled  DerivativeFilterVariant=ForwardEulerFilter  NVariant=InternalParameters  NCopyVariant=Disabled  FilterICVariant=InternalICsFilter  IntegratorICVariant=InternalICs  ExternalResetVariant=Disabled  TRSumVariant=Passthrough  SumFdbkVariant=Disabled  SumVariant=Sum_PID  TsampFilterVariant=InternalTs  TsampNgainVariant=Passthrough  TsampIntegralVariant=Passthrough  ExternalSaturationOutDataTypeStr=Inherit: Same as second input
  PWM7 : simulink/Discontinuities/PWM  DisableCoverage=on  Period=2  InitialDelay=0  DisallowZeroDutyCycle=off  RunAtFixedTimeIntervals=off  SampleTime=0.1
  PWM8 : simulink/Discontinuities/PWM  DisableCoverage=on  Period=2  InitialDelay=0  DisallowZeroDutyCycle=off  RunAtFixedTimeIntervals=off  SampleTime=0.1
  Saturation13 : Saturate  UpperLimit=1  LowerLimit=0
  Saturation14 : Saturate  UpperLimit=1  LowerLimit=0
  Sum6 : Sum  Inputs=|+-
  Output : Outport
  wires:
  PID Controller5/1 -> Gain4/1, Saturation14/1
  Saturation13/1 -> PWM8/1
  Gain4/1 -> Saturation13/1
  Constant/1 -> Sum6/1
  Sum6/1 -> PID Controller5/1
  Saturation14/1 -> PWM7/1
  PWM8/1 -> Mux/2
  PWM7/1 -> Mux/1
  Mux/1 -> Output/1
  Input/1 -> Sum6/2

== system StateFlow_varB/Subsystem6/Subsystem/Subsystem12 ==
  Input : Inport
  Enable : EnablePort
  Constant : Constant  Value=s  OutDataTypeStr=Bus: s_bus
  Constant1 : Constant  Value=Desired_pressure_in_oxidiser_tank
  MATLAB Function2 : MATLAB Function  TreatAsAtomicUnit=on
  Mux : Mux  Inputs=2
  PWM1 : simulink/Discontinuities/PWM  DisableCoverage=on  Period=2.5  InitialDelay=0  DisallowZeroDutyCycle=off  RunAtFixedTimeIntervals=off  SampleTime=0.1
  PWM2 : simulink/Discontinuities/PWM  DisableCoverage=on  Period=2.5  InitialDelay=0  DisallowZeroDutyCycle=off  RunAtFixedTimeIntervals=off  SampleTime=0.1
  Sum10 : Sum  Inputs=|+-
  Unit Delay : UnitDelay  InitialCondition=0.1  SampleTime=-1  HasFrameUpgradeWarning=on
  Unit Delay1 : UnitDelay  InitialCondition=Desired_pressure_in_oxidiser_tank-1  SampleTime=-1  HasFrameUpgradeWarning=on
  Output : Outport
  wires:
  Constant1/1 -> Sum10/1
  Sum10/1 -> Unit Delay1/1, MATLAB Function2/1(u)
  Constant/1 -> MATLAB Function2/3(workspace)
  Mux/1 -> Output/1
  Input/1 -> Sum10/2
  MATLAB Function2/3(duty) -> Unit Delay/1
  Unit Delay/1 -> MATLAB Function2/4(previous_duty)
  PWM1/1 -> Mux/1
  MATLAB Function2/1(fill) -> PWM1/1
  MATLAB Function2/2(release) -> PWM2/1
  PWM2/1 -> Mux/2
  Unit Delay1/1 -> MATLAB Function2/2(prev_u)

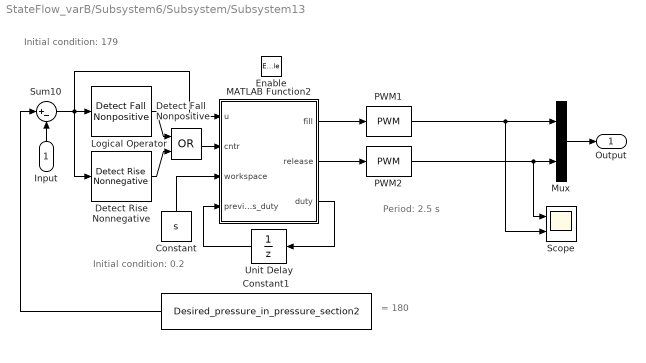
== system StateFlow_varB/Subsystem6/Subsystem/Subsystem13 ==
  note: Initial condition: 179
  note: Period: 2.5 s
  note: Initial condition: 0.2
  note: = 180
  Input : Inport
  Enable : EnablePort  StatesWhenEnabling=reset
  Constant : Constant  Value=s  OutDataTypeStr=Bus: s_bus
  Constant1 : Constant  Value=Desired_pressure_in_pressure_section2
  Detect Fall Nonpositive : simulink/Logic and Bit Operations/Detect Fall Nonpositive  vinit=Desired_pressure_in_pressure_section2 - 1  OutDataTypeStr=boolean
  Detect Rise Nonnegative : simulink/Logic and Bit Operations/Detect Rise Nonnegative  vinit=Desired_pressure_in_pressure_section2-1  OutDataTypeStr=boolean
  Logical Operator : Logic  Operator=OR  AllPortsSameDT=off  OutDataTypeStr=boolean
  MATLAB Function2 : MATLAB Function  TreatAsAtomicUnit=on
  Mux : Mux  Inputs=2
  PWM1 : simulink/Discontinuities/PWM  DisableCoverage=on  Period=2.5  InitialDelay=0  DisallowZeroDutyCycle=off  RunAtFixedTimeIntervals=off  SampleTime=0.1
  PWM2 : simulink/Discontinuities/PWM  DisableCoverage=on  Period=2.5  InitialDelay=0  DisallowZeroDutyCycle=off  RunAtFixedTimeIntervals=off  SampleTime=0.1
  Scope : Scope  NumInputPorts=2
  Sum10 : Sum  Inputs=|+-
  Unit Delay : UnitDelay  InitialCondition=0.2  SampleTime=-1  HasFrameUpgradeWarning=on
  Output : Outport
  wires:
  Logical Operator/1 -> MATLAB Function2/2(cntr)
  Detect Fall Nonpositive/1 -> Logical Operator/1
  Detect Rise Nonnegative/1 -> Logical Operator/2
  PWM2/1 -> Scope/1, Mux/2
  MATLAB Function2/2(release) -> PWM2/1
  MATLAB Function2/1(fill) -> PWM1/1
  PWM1/1 -> Scope/2, Mux/1
  Unit Delay/1 -> MATLAB Function2/4(previous_duty)
  MATLAB Function2/3(duty) -> Unit Delay/1
  Input/1 -> Sum10/2
  Mux/1 -> Output/1
  Constant/1 -> MATLAB Function2/3(workspace)
  Sum10/1 -> Detect Fall Nonpositive/1, MATLAB Function2/1(u), Detect Rise Nonnegative/1
  Constant1/1 -> Sum10/1

== system StateFlow_varB/Subsystem6/Subsystem/Subsystem14 ==
  Input : Inport
  Enable : EnablePort
  Constant : Constant  Value=Desired_pressure_in_oxidiser_tank
  Constant1 : Constant  Commented=on  Value=s  OutDataTypeStr=Bus: s_bus
  Gain5 : Gain  Gain=-1
  MATLAB Function : MATLAB Function  Commented=on  TreatAsAtomicUnit=on
  Mux : Mux  Inputs=2
  PID Controller7 : slpidlib/PID Controller  Controller=PID  Form=Parallel  TimeDomain=Discrete-time  UseExternalTs=off  SampleTime=-1  IntegratorMethod=Forward Euler  FilterMethod=Forward Euler  ControllerParametersSource=internal  P=0.008  I=0.00068  UseKiTs=off  D=0  N=0  UseFilter=on  TunerSelectOption=Transfer Function Based (PID Tuner App)  InitialConditionSource=internal  InitialConditionForIntegrator=0  InitialConditionForFilter=0  DifferentiatorICPrevScaledInput=0  ExternalReset=none  TrackingMode=off  Kt=1  LimitOutput=on  SatLimitsSource=internal  UpperSaturationLimit=1  LowerSaturationLimit=-1  LinearizeAsGain=off  AntiWindupMode=clamping  Kb=1  LimitIntegrator=on  UpperIntegratorSaturationLimit=1  LowerIntegratorSaturationLimit=-1  POutMin=[]  POutMax=[]  IOutMin=[]  IOutMax=[]  DOutMin=[]  DOutMax=[]  NOutMin=[]  NOutMax=[]  SumOutMin=[]  SumOutMax=[]  SaturationOutMin=[]  SaturationOutMax=[]  PParamMin=[]  PParamMax=[]  IParamMin=[]  IParamMax=[]  DParamMin=[]  DParamMax=[]  NParamMin=[]  NParamMax=[]  KbParamMin=[]  KbParamMax=[]  KtParamMin=[]  KtParamMax=[]  KbOutMin=[]  KbOutMax=[]  KtOutMin=[]  KtOutMax=[]  IntegratorOutMin=[]  IntegratorOutMax=[]  FilterOutMin=[]  FilterOutMax=[]  SumI1OutMin=[]  SumI1OutMax=[]  SumI2OutMin=[]  SumI2OutMax=[]  SumI3OutMin=[]  SumI3OutMax=[]  SumI4OutMin=[]  SumI4OutMax=[]  SumDOutMin=[]  SumDOutMax=[]  DifferentiatorOutMin=[]  DifferentiatorOutMax=[]  FilterDiffOutCoefMin=[]  FilterDiffOutCoefMax=[]  ReciprocalOutMin=[]  ReciprocalOutMax=[]  SumDenOutMin=[]  SumDenOutMax=[]  SumNumOutMin=[]  SumNumOutMax=[]  DivideOutMin=[]  DivideOutMax=[]  UdiffTsProdOutMin=[]  UdiffTsProdOutMax=[]  NTsProdOutMin=[]  NTsProdOutMax=[]  UintegralTsProdOutMin=[]  UintegralTsProdOutMax=[]  UngainTsProdOutMin=[]  UngainTsProdOutMax=[]  ClampingZeroOutDataTypeStr=Inherit: Inherit via back propagation  ClampingZeroOutMin=[]  ClampingZeroOutMax=[]  FilterDenConstantOutDataTypeStr=Inherit: Inherit via back propagation  FilterDenConstantOutMin=[]  FilterDenConstantOutMax=[]  PCopyOutDataTypeStr=Inherit: Inherit via back propagation  PCopyOutMin=[]  PCopyOutMax=[]  NCopyOutDataTypeStr=Inherit: Inherit via back propagation  NCopyOutMin=[]  NCopyOutMax=[]  IntegratorContinuousStateAttributes=''  IntegratorStateMustResolveToSignalObject=off  IntegratorRTWStateStorageClass=Auto  FilterContinuousStateAttributes=''  FilterStateMustResolveToSignalObject=off  FilterRTWStateStorageClass=Auto  ParallelPVariant=InternalParameters  IdealPVariant=Disabled  IVariant=InternalParameters  DVariant=InternalParameters  IntegratorVariant=Discrete  SatVariant=Enabled  AWVariant=DiscClampingParallel  PCopyVariant=Disabled  TRVariant=Disabled  FdbkBlocksVariant=Forward  IdealPFdbkVariant=Disabled  SatFdbkVariant=Disabled  DerivativeFilterVariant=ForwardEulerFilter  NVariant=InternalParameters  NCopyVariant=Disabled  FilterICVariant=InternalICsFilter  IntegratorICVariant=InternalICs  ExternalResetVariant=Disabled  TRSumVariant=Passthrough  SumFdbkVariant=Disabled  SumVariant=Sum_PID  TsampFilterVariant=InternalTs  TsampNgainVariant=Passthrough  TsampIntegralVariant=Passthrough  ExternalSaturationOutDataTypeStr=Inherit: Same as second input
  PWM : simulink/Discontinuities/PWM  DisableCoverage=on  Period=2  InitialDelay=0  DisallowZeroDutyCycle=off  RunAtFixedTimeIntervals=off  SampleTime=0.1
  PWM1 : simulink/Discontinuities/PWM  DisableCoverage=on  Period=2  InitialDelay=0  DisallowZeroDutyCycle=off  RunAtFixedTimeIntervals=off  SampleTime=0.1
  Sum9 : Sum  Inputs=|+-
  Terminator : Terminator  Commented=on
  Output : Outport
  wires:
  Constant/1 -> Sum9/1
  Sum9/1 -> PID Controller7/1
  PID Controller7/1 -> PWM/1, Gain5/1
  PWM/1 -> Mux/1
  Gain5/1 -> PWM1/1
  Input/1 -> Sum9/2
  Mux/1 -> Output/1
  MATLAB Function/1(y) -> Terminator/1
  Constant1/1 -> MATLAB Function/3(workspace)
  PWM1/1 -> Mux/2

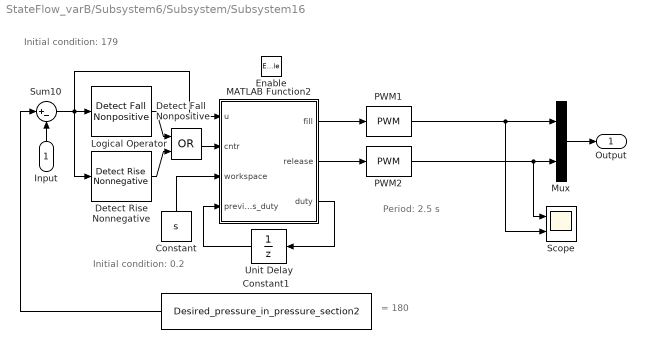
== system StateFlow_varB/Subsystem6/Subsystem/Subsystem16 ==
  note: Initial condition: 179
  note: Period: 2.5 s
  note: Initial condition: 0.2
  note: = 180
  Input : Inport
  Enable : EnablePort  StatesWhenEnabling=reset
  Constant : Constant  Value=s  OutDataTypeStr=Bus: s_bus
  Constant1 : Constant  Value=Desired_pressure_in_pressure_section2
  Detect Fall Nonpositive : simulink/Logic and Bit Operations/Detect Fall Nonpositive  vinit=Desired_pressure_in_pressure_section2 - 1  OutDataTypeStr=boolean
  Detect Rise Nonnegative : simulink/Logic and Bit Operations/Detect Rise Nonnegative  vinit=Desired_pressure_in_pressure_section2-1  OutDataTypeStr=boolean
  Logical Operator : Logic  Operator=OR  AllPortsSameDT=off  OutDataTypeStr=boolean
  MATLAB Function2 : MATLAB Function  TreatAsAtomicUnit=on
  Mux : Mux  Inputs=2
  PWM1 : simulink/Discontinuities/PWM  DisableCoverage=on  Period=2.5  InitialDelay=0  DisallowZeroDutyCycle=off  RunAtFixedTimeIntervals=off  SampleTime=0.1
  PWM2 : simulink/Discontinuities/PWM  DisableCoverage=on  Period=2.5  InitialDelay=0  DisallowZeroDutyCycle=off  RunAtFixedTimeIntervals=off  SampleTime=0.1
  Scope : Scope  NumInputPorts=2
  Sum10 : Sum  Inputs=|+-
  Unit Delay : UnitDelay  InitialCondition=0.2  SampleTime=-1  HasFrameUpgradeWarning=on
  Output : Outport
  wires:
  Logical Operator/1 -> MATLAB Function2/2(cntr)
  Detect Fall Nonpositive/1 -> Logical Operator/1
  Detect Rise Nonnegative/1 -> Logical Operator/2
  PWM2/1 -> Scope/1, Mux/2
  MATLAB Function2/2(release) -> PWM2/1
  MATLAB Function2/1(fill) -> PWM1/1
  PWM1/1 -> Scope/2, Mux/1
  Unit Delay/1 -> MATLAB Function2/4(previous_duty)
  MATLAB Function2/3(duty) -> Unit Delay/1
  Input/1 -> Sum10/2
  Mux/1 -> Output/1
  Constant/1 -> MATLAB Function2/3(workspace)
  Sum10/1 -> Detect Fall Nonpositive/1, MATLAB Function2/1(u), Detect Rise Nonnegative/1
  Constant1/1 -> Sum10/1

== system StateFlow_varB/Subsystem6/Subsystem/Subsystem18 ==
  note: Initial condition: 149
  note: Period: 2.5 s
  note: Initial condition: 0.2
  note: = 150
  Input : Inport
  Enable : EnablePort  StatesWhenEnabling=reset
  Constant : Constant  Value=s  OutDataTypeStr=Bus: s_bus
  Constant1 : Constant  Value=Desired_pressure_in_pressure_section1
  Detect Fall Nonpositive : simulink/Logic and Bit Operations/Detect Fall Nonpositive  vinit=Desired_pressure_in_pressure_section1-1  OutDataTypeStr=boolean
  Detect Rise Nonnegative : simulink/Logic and Bit Operations/Detect Rise Nonnegative  vinit=Desired_pressure_in_pressure_section1-1  OutDataTypeStr=boolean
  Logical Operator : Logic  Operator=OR  AllPortsSameDT=off  OutDataTypeStr=boolean
  MATLAB Function2 : MATLAB Function  TreatAsAtomicUnit=on
  Mux : Mux  Inputs=2
  PWM1 : simulink/Discontinuities/PWM  DisableCoverage=on  Period=2.5  InitialDelay=0  DisallowZeroDutyCycle=off  RunAtFixedTimeIntervals=off  SampleTime=0.1
  PWM2 : simulink/Discontinuities/PWM  DisableCoverage=on  Period=2.5  InitialDelay=0  DisallowZeroDutyCycle=off  RunAtFixedTimeIntervals=off  SampleTime=0.1
  Sum10 : Sum  Inputs=|+-
  Unit Delay : UnitDelay  InitialCondition=0.2  SampleTime=-1  HasFrameUpgradeWarning=on
  Output : Outport
  wires:
  Logical Operator/1 -> MATLAB Function2/2(cntr)
  Detect Fall Nonpositive/1 -> Logical Operator/1
  Detect Rise Nonnegative/1 -> Logical Operator/2
  PWM2/1 -> Mux/2
  MATLAB Function2/2(release) -> PWM2/1
  MATLAB Function2/1(fill) -> PWM1/1
  PWM1/1 -> Mux/1
  Unit Delay/1 -> MATLAB Function2/4(previous_duty)
  MATLAB Function2/3(duty) -> Unit Delay/1
  Input/1 -> Sum10/2
  Mux/1 -> Output/1
  Constant/1 -> MATLAB Function2/3(workspace)
  Sum10/1 -> Detect Fall Nonpositive/1, MATLAB Function2/1(u), Detect Rise Nonnegative/1
  Constant1/1 -> Sum10/1

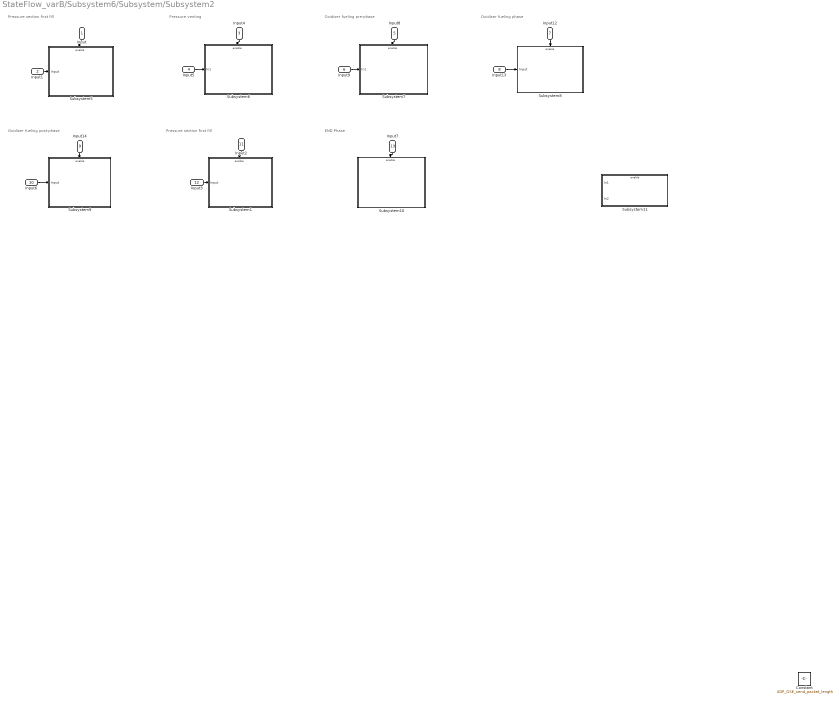
== system StateFlow_varB/Subsystem6/Subsystem/Subsystem2 ==
  note: END Phase
  note: Oxidiser fueling phase
  note: Pressure venting
  note: Pressure section first fill
  note: Oxidiser fueling pre-phase
  note: Oxidiser fueling post-phase
  note: Pressure section first fill
  Input : Inport
  Input1 : Inport  Port=2
  Input4 : Inport  Port=3
  Input5 : Inport  Port=4
  Input8 : Inport  Port=5
  Input9 : Inport  Port=6
  Input12 : Inport  Port=7
  Input13 : Inport  Port=8
  Input14 : Inport  Port=9
  Input6 : Inport  Port=10
  Input2 : Inport  Port=11
  Input3 : Inport  Port=12
  Input7 : Inport  Port=13
  Constant : Constant  Value=UDP_GSE_send_packet_length
  Subsystem1 : Subsystem
  Subsystem10 : Subsystem
  Subsystem11 : Subsystem
  Subsystem5 : Subsystem
  Subsystem6 : Subsystem
  Subsystem7 : Subsystem
  Subsystem8 : Subsystem
  Subsystem9 : Subsystem
  wires:
  Input/1 -> Subsystem5/Enable
  Input1/1 -> Subsystem5/1(Input)
  Input4/1 -> Subsystem6/Enable
  Input5/1 -> Subsystem6/1(In1)
  Input8/1 -> Subsystem7/Enable
  Input9/1 -> Subsystem7/1(In1)
  Input12/1 -> Subsystem8/Enable
  Input13/1 -> Subsystem8/1(Input)
  Input14/1 -> Subsystem9/Enable
  Input6/1 -> Subsystem9/1(Input)
  Input7/1 -> Subsystem10/Enable
  Input3/1 -> Subsystem1/1(Input)
  Input2/1 -> Subsystem1/Enable

== system StateFlow_varB/Subsystem6/Subsystem/Subsystem3 ==
  note: Period: 2 s
  note: Proportional (P): 0.008
  note: Saturation - Upper limit: 1
  note: Saturation - Lower limit: -1
  note: = 150
  Input : Inport
  Enable : EnablePort  StatesWhenEnabling=reset
  Constant : Constant  Value=Desired_pressure_in_pressure_section1
  Gain6 : Gain  Gain=-1
  Mux : Mux  Inputs=2
  PID Controller4 : slpidlib/PID Controller  Controller=P  Form=Parallel  TimeDomain=Discrete-time  UseExternalTs=off  SampleTime=-1  IntegratorMethod=Forward Euler  FilterMethod=Forward Euler  ControllerParametersSource=internal  P=0.008  I=0.01  UseKiTs=off  D=0  N=100  UseFilter=on  TunerSelectOption=Transfer Function Based (PID Tuner App)  InitialConditionSource=internal  InitialConditionForIntegrator=0  InitialConditionForFilter=0  DifferentiatorICPrevScaledInput=0  ExternalReset=none  TrackingMode=off  Kt=1  LimitOutput=on  SatLimitsSource=internal  UpperSaturationLimit=1  LowerSaturationLimit=-1  LinearizeAsGain=on  AntiWindupMode=none  Kb=1  LimitIntegrator=on  UpperIntegratorSaturationLimit=150  LowerIntegratorSaturationLimit=-inf  POutMin=[]  POutMax=[]  IOutMin=[]  IOutMax=[]  DOutMin=[]  DOutMax=[]  NOutMin=[]  NOutMax=[]  SumOutMin=[]  SumOutMax=[]  SaturationOutMin=[]  SaturationOutMax=[]  PParamMin=[]  PParamMax=[]  IParamMin=[]  IParamMax=[]  DParamMin=[]  DParamMax=[]  NParamMin=[]  NParamMax=[]  KbParamMin=[]  KbParamMax=[]  KtParamMin=[]  KtParamMax=[]  KbOutMin=[]  KbOutMax=[]  KtOutMin=[]  KtOutMax=[]  IntegratorOutMin=[]  IntegratorOutMax=[]  FilterOutMin=[]  FilterOutMax=[]  SumI1OutMin=[]  SumI1OutMax=[]  SumI2OutMin=[]  SumI2OutMax=[]  SumI3OutMin=[]  SumI3OutMax=[]  SumI4OutMin=[]  SumI4OutMax=[]  SumDOutMin=[]  SumDOutMax=[]  DifferentiatorOutMin=[]  DifferentiatorOutMax=[]  FilterDiffOutCoefMin=[]  FilterDiffOutCoefMax=[]  ReciprocalOutMin=[]  ReciprocalOutMax=[]  SumDenOutMin=[]  SumDenOutMax=[]  SumNumOutMin=[]  SumNumOutMax=[]  DivideOutMin=[]  DivideOutMax=[]  UdiffTsProdOutMin=[]  UdiffTsProdOutMax=[]  NTsProdOutMin=[]  NTsProdOutMax=[]  UintegralTsProdOutMin=[]  UintegralTsProdOutMax=[]  UngainTsProdOutMin=[]  UngainTsProdOutMax=[]  ClampingZeroOutDataTypeStr=Inherit: Inherit via back propagation  ClampingZeroOutMin=[]  ClampingZeroOutMax=[]  FilterDenConstantOutDataTypeStr=Inherit: Inherit via back propagation  FilterDenConstantOutMin=[]  FilterDenConstantOutMax=[]  PCopyOutDataTypeStr=Inherit: Inherit via back propagation  PCopyOutMin=[]  PCopyOutMax=[]  NCopyOutDataTypeStr=Inherit: Inherit via back propagation  NCopyOutMin=[]  NCopyOutMax=[]  IntegratorContinuousStateAttributes=''  IntegratorStateMustResolveToSignalObject=off  IntegratorRTWStateStorageClass=Auto  FilterContinuousStateAttributes=''  FilterStateMustResolveToSignalObject=off  FilterRTWStateStorageClass=Auto  ParallelPVariant=InternalParameters  IdealPVariant=Disabled  IVariant=Disabled  DVariant=Disabled  IntegratorVariant=Disabled  SatVariant=Enabled  AWVariant=Disabled  PCopyVariant=Disabled  TRVariant=Disabled  FdbkBlocksVariant=Forward  IdealPFdbkVariant=Disabled  SatFdbkVariant=Disabled  DerivativeFilterVariant=Disabled  NVariant=Disabled  NCopyVariant=Disabled_SignalSpec  FilterICVariant=Disabled  IntegratorICVariant=Disabled  ExternalResetVariant=Disabled  TRSumVariant=Passthrough  SumFdbkVariant=Disabled  SumVariant=Passthrough_P  TsampFilterVariant=InternalTs  TsampNgainVariant=Passthrough  TsampIntegralVariant=Disabled_SignalSpec  ExternalSaturationOutDataTypeStr=Inherit: Same as second input
  PWM12 : simulink/Discontinuities/PWM  DisableCoverage=on  Period=2  InitialDelay=0  DisallowZeroDutyCycle=off  RunAtFixedTimeIntervals=off  SampleTime=0.1
  PWM6 : simulink/Discontinuities/PWM  DisableCoverage=on  Period=2  InitialDelay=0  DisallowZeroDutyCycle=off  RunAtFixedTimeIntervals=off  SampleTime=0.1
  Scope : Scope  NumInputPorts=3
  Sum4 : Sum  Inputs=|+-
  Output : Outport
  wires:
  PID Controller4/1 -> PWM6/1, Scope/3, Gain6/1
  Gain6/1 -> PWM12/1
  Mux/1 -> Output/1
  PWM6/1 -> Scope/2, Mux/1
  PWM12/1 -> Scope/1, Mux/2
  Constant/1 -> Sum4/1
  Input/1 -> Sum4/2
  Sum4/1 -> PID Controller4/1

== system StateFlow_varB/Subsystem6/Subsystem/Subsystem4 ==
  Input : Inport
  Enable : EnablePort
  Constant : Constant  Value=Desired_pressure_in_pressure_section1
  Dead Zone1 : DeadZone  LowerValue=-Acceptable_press_offset  UpperValue=Acceptable_press_offset  SaturateOnIntegerOverflow=off
  Gain2 : Gain  Gain=-1
  Mux : Mux  Inputs=2
  Relay1 : Relay  OnSwitchValue=Acceptable_press_offset  OffSwitchValue=0
  Relay2 : Relay  OnSwitchValue=Acceptable_press_offset  OffSwitchValue=0
  Sum5 : Sum  Inputs=|+-
  Output : Outport
  wires:
  Sum5/1 -> Dead Zone1/1
  Relay1/1 -> Mux/1
  Dead Zone1/1 -> Relay1/1, Gain2/1
  Gain2/1 -> Relay2/1
  Constant/1 -> Sum5/1
  Relay2/1 -> Mux/2
  Input/1 -> Sum5/2
  Mux/1 -> Output/1
